simulink model "matlabfunction_block"  (R2022b)
settings: Solver=FixedStepAuto  StartTime=0.0  StopTime=10.0  FixedStep=0.01  RelTol=1e-3
settings Model: Creator=Brigosha_Guest  LastModifiedBy=Brigosha_Guest

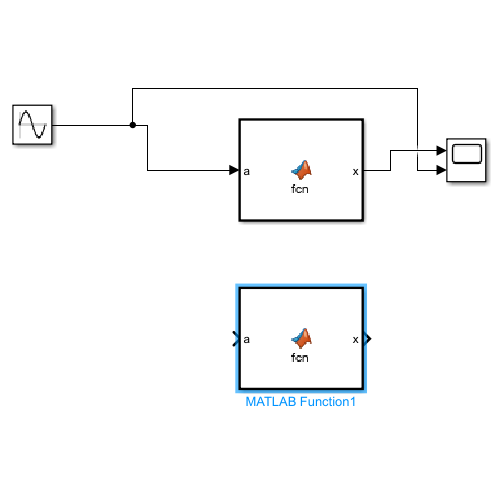
[thumbnail: Simulink's stored preview of the top-level diagram]
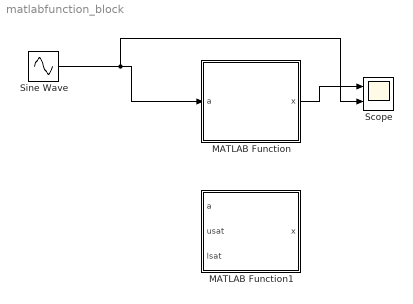
== system matlabfunction_block ==
  MATLAB Function : MATLAB Function  TreatAsAtomicUnit=on
  MATLAB Function1 : MATLAB Function  TreatAsAtomicUnit=on
  Scope : Scope  NumInputPorts=2
  Sine Wave : Sin  SampleTime=0
  wires:
  Sine Wave/1 -> Scope/2, MATLAB Function/1(a)
  MATLAB Function/1(x) -> Scope/1

== matlab function matlabfunction_block/MATLAB Function1 ==
  data: x output; a input; usat input; lsat input
function x = fcn(a,usat,lsat)
if a>=usat
    x=usat;
elseif a<=lsat
        x=lsat;
else
    x=a;
end

== matlab function matlabfunction_block/MATLAB Function ==
  data: x output; a input
function x = fcn(a)
if a>=0.5
    x=0.5;
elseif a<=-0.5
        x=-0.5;
else
    x=a;
end
